simulink model "Test_N2"  (R2022a)
settings: Solver=ode3  StartTime=0.0  StopTime=inf  FixedStep=0.05  RelTol=1e-3
libraries: EcBlockToolbox x1, Utilities x1

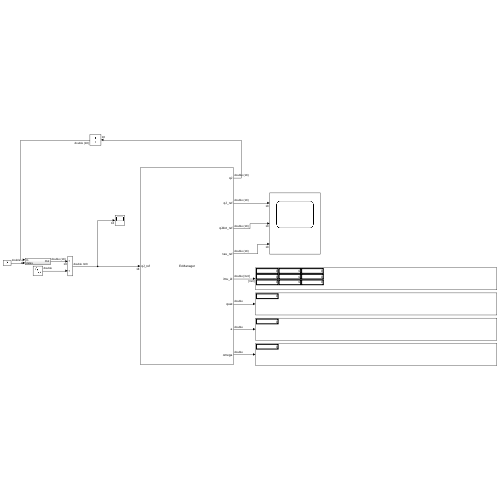
[thumbnail: Simulink's stored preview of the top-level diagram]
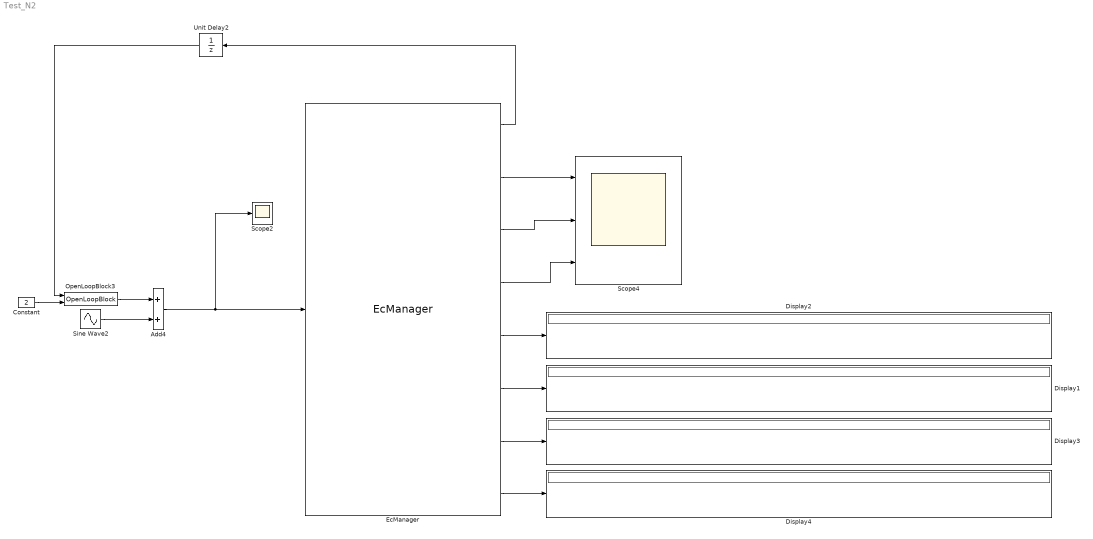
== system Test_N2 ==
  Add4 : Sum
  Constant : Constant  Value=2
  Display{1..4} (4 alike) : Display
  EcManager : EcBlockToolbox/EcManager  ReadingsList={'qJ', 'qJ_ref', 'qJdot_ref', 'tau_ref'}  ReferencesList={'qJ_ref'}  ImuList={'imu_id', 'quat', 'a', 'omega'}
  OpenLoopBlock3 : Utilities/OpenLoopBlock  SystemSampleTime=-1  VariantActivationTime=update diagram  Latency=0  AutoFrameSizeCalculation=off
  Scope2 : Scope
  Scope4 : Scope  NumInputPorts=3
  Sine Wave2 : Sin  Amplitude=5  SampleTime=0
  Unit Delay2 : UnitDelay  SampleTime=-1  HasFrameUpgradeWarning=on
  wires:
  OpenLoopBlock3/1 -> Add4/1
  Constant/1 -> OpenLoopBlock3/2
  Add4/1 -> Scope2/1, EcManager/1
  Sine Wave2/1 -> Add4/2
  Unit Delay2/1 -> OpenLoopBlock3/1
  EcManager/8 -> Display4/1
  EcManager/4 -> Scope4/3
  EcManager/1 -> Unit Delay2/1
  EcManager/2 -> Scope4/1
  EcManager/3 -> Scope4/2
  EcManager/5 -> Display2/1
  EcManager/6 -> Display1/1
  EcManager/7 -> Display3/1
